simulink model "boost_conv_try2"  (R2023a)
settings: Solver=ode15s  StartTime=0.0  StopTime=0.1  MaxStep=1e-8  RelTol=1e-6  AbsTol=1e-6
settings Model: Creator=gabrielcrisan  LastModifiedBy=gabrielcrisan

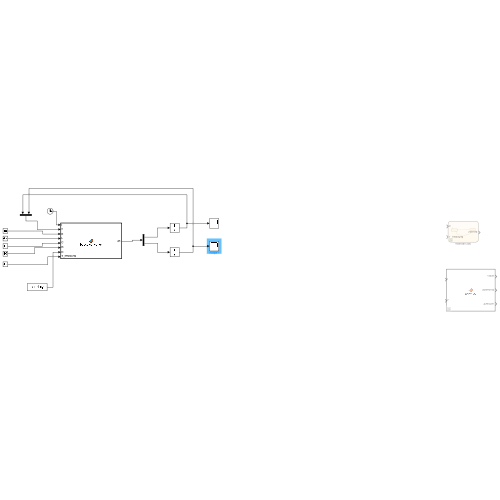
[thumbnail: Simulink's stored preview of the top-level diagram]
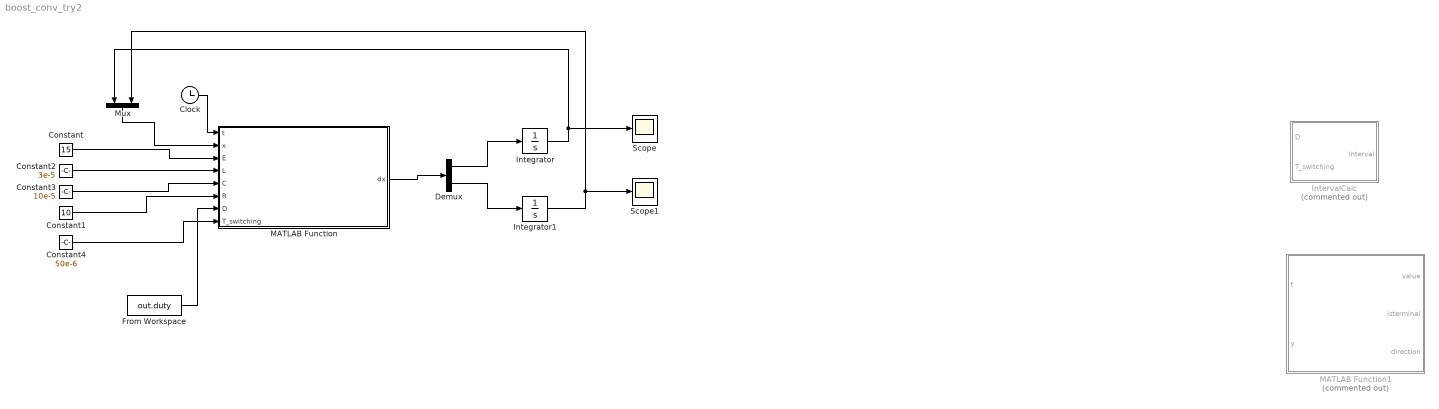
== system boost_conv_try2 ==
  Clock : Clock
  Constant : Constant  Value=15
  Constant1 : Constant  Value=10
  Constant2 : Constant  Value=3e-5
  Constant3 : Constant  Value=10e-5
  Constant4 : Constant  Value=50e-6
  Demux : Demux  Outputs=2
  From Workspace : FromWorkspace  VariableName=out.duty
  Integrator : Integrator
  Integrator1 : Integrator
  IntervalCalc : Stateflow chart  Commented=on  TreatAsAtomicUnit=on
  MATLAB Function : MATLAB Function  TreatAsAtomicUnit=on
  MATLAB Function1 : MATLAB Function  Commented=on  TreatAsAtomicUnit=on
  Mux : Mux  Inputs=2
  Scope : Scope
  Scope1 : Scope
  wires:
  MATLAB Function/1(dx) -> Demux/1
  Demux/1 -> Integrator/1
  Demux/2 -> Integrator1/1
  Constant/1 -> MATLAB Function/3(E)
  Constant1/1 -> MATLAB Function/6(R)
  Constant2/1 -> MATLAB Function/4(L)
  Constant3/1 -> MATLAB Function/5(C)
  Integrator/1 -> Scope/1, Mux/1
  Integrator1/1 -> Scope1/1, Mux/2
  Mux/1 -> MATLAB Function/2(x)
  Clock/1 -> MATLAB Function/1(t)
  Constant4/1 -> MATLAB Function/8(T_switching)
  From Workspace/1 -> MATLAB Function/7(D)

== matlab function boost_conv_try2/MATLAB Function1 ==
  data: t input; value output; y input; isterminal output; direction output
function [value, isterminal, direction] = conv_ev(t, y)
    value = y(1);  % detect iL = 0
    isterminal = 1;  % stop the integration
    direction = -1;  % negative direction
end

== matlab function boost_conv_try2/MATLAB Function ==
  data: t input; dx output; x input; E input; L input; C input; R input; D input; T_switching input
function dx = boost_converter(t, x, E, L, C, R, D, T_switching)
    % States
    iL = x(1);  
    uC = x(2);  

    % Calculate current interval
    t_mod = mod(t, T_switching);
    if t_mod < D * T_switching
        interval = 1;  % Switch is on
    else
        interval = 2;  % Switch is off
    end

    % Calculate derivatives based on interval
    if interval == 1
        diL_dt = E / L;
        duC_dt = -uC / (R * C);
    elseif interval == 2
        diL_dt = (E - uC) / L;
        duC_dt = (iL - uC / R) / C;
    else
        diL_dt = 0;
        duC_dt = 0;
    end

    % Output derivatives
    dx = [diL_dt; duC_dt];
end

== stateflow chart boost_conv_try2/IntervalCalc ==
  state SwitchOff
    entry: interval = 2;
  state SwitchOn
    entry: interval = 1;
  (default) -> SwitchOn
  SwitchOn -> SwitchOff : [after(D * T_switching, sec)]
  SwitchOff -> SwitchOn : [after((1-D) * T_switching, sec)]
  data: D input; T_switching input; interval output
